simulink model "FH_SS"  (R2018b)
settings: Solver=ode5  StartTime=0.0  StopTime=N*Tb  FixedStep=Tsampling  RelTol=1e-3
values from neighbouring files (symbols this model uses):
  Eb = 2    [FH_Script.m]
  Tb = 1/100    (= 0.01)    [FH_Script.m]
  Tc = Tb/(MultPer*Nchips)    (= 0.000285714285714)    [FH_Script.m]
libraries: dsparch4 x5, commsynccomp2 x4, commrandsrc3 x1, simulink x1
settings Model: Creator=lukit  LastModifiedBy=lukit

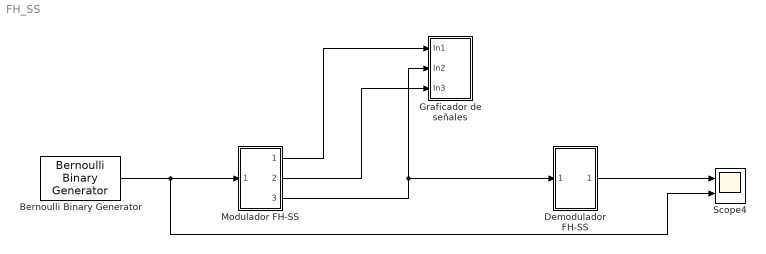
== system FH_SS ==
  Bernoulli Binary Generator : commrandsrc3/Bernoulli Binary Generator  ProbabilityOfZero=0.5  SeedSource=Auto  Seed=0  SampleTime=Tb  SamplesPerFrame=1  OutputDataType=double  SimulateUsing=Interpreted execution
  Demodulador FH-SS : Subsystem
  Graficador de señales : Subsystem
  Modulador FH-SS : Subsystem
  Scope4 : Scope  NumInputPorts=2
  wires:
  Modulador FH-SS/3(Out3) -> Demodulador FH-SS/1(In1), Graficador de señales/2(In2)
  Bernoulli Binary Generator/1 -> Scope4/2, Modulador FH-SS/1(In1)
  Modulador FH-SS/1(Out1) -> Graficador de señales/1(In1)
  Modulador FH-SS/2(Out2) -> Graficador de señales/3(In3)
  Demodulador FH-SS/1(Out1) -> Scope4/1

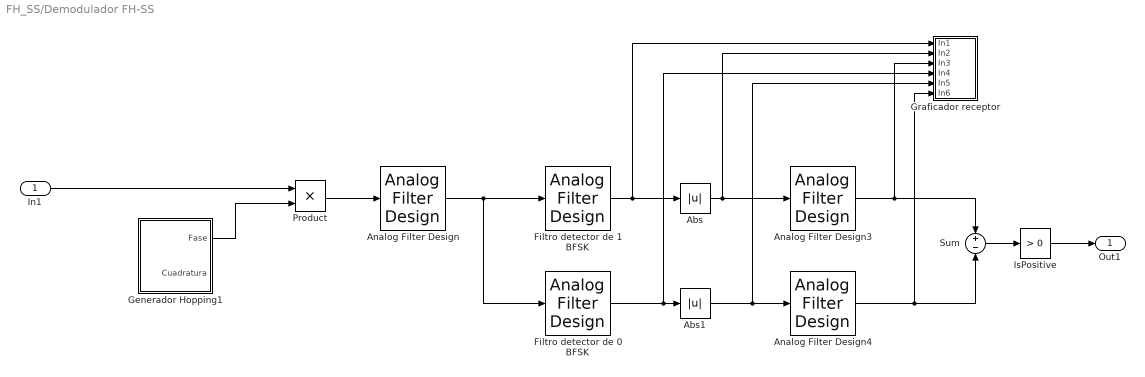
== system FH_SS/Demodulador FH-SS ==
  In1 : Inport
  Abs : Abs
  Abs1 : Abs
  Analog Filter Design : dsparch4/Analog Filter Design  method=Butterworth  filttype=Bandpass  N=8  Wlo=2*pi*(2*(1/Tc) - (1/Tc))  Whi=2*pi*(4*(1/Tc) +(1/Tc))  Rp=2  Rs=40
  Analog Filter Design3 : dsparch4/Analog Filter Design  method=Butterworth  filttype=Lowpass  N=8  Wlo=2*pi*((1/Tc))  Whi=2*pi*((2*(1/Tc)) +(1/Tc))  Rp=2  Rs=40
  Analog Filter Design4 : dsparch4/Analog Filter Design  method=Butterworth  filttype=Lowpass  N=8  Wlo=2*pi*((1/Tc))  Whi=2*pi*((2*(1/Tc)) +(1/Tc))  Rp=2  Rs=40
  Filtro detector de 0 BFSK : dsparch4/Analog Filter Design  method=Butterworth  filttype=Bandpass  N=8  Wlo=2*pi*((4*(1/Tc)) - (1/Tc))  Whi=2*pi*((4*(1/Tc)) +(1/Tc))  Rp=2  Rs=40
  Filtro detector de 1 BFSK : dsparch4/Analog Filter Design  method=Butterworth  filttype=Bandpass  N=8  Wlo=2*pi*((2*(1/Tc)) - (1/Tc))  Whi=2*pi*((2*(1/Tc)) +(1/Tc))  Rp=2  Rs=40
  Generador Hopping1 : Subsystem
  Graficador receptor : Subsystem
  IsPositive : simulink/Logic and Bit Operations/Compare To Zero  relop=>  OutDataTypeStr=boolean
  Product : Product
  Sum : Sum  Inputs=+-
  Out1 : Outport
  wires:
  Product/1 -> Analog Filter Design/1
  Analog Filter Design3/1 -> Sum/1, Graficador receptor/3(In3)
  Abs/1 -> Analog Filter Design3/1, Graficador receptor/2(In2)
  Filtro detector de 1 BFSK/1 -> Abs/1, Graficador receptor/1(In1)
  Generador Hopping1/1(Fase) -> Product/2
  Analog Filter Design/1 -> Filtro detector de 0 BFSK/1, Filtro detector de 1 BFSK/1
  Analog Filter Design4/1 -> Sum/2, Graficador receptor/6(In6)
  Filtro detector de 0 BFSK/1 -> Graficador receptor/4(In4), Abs1/1
  Abs1/1 -> Graficador receptor/5(In5), Analog Filter Design4/1
  In1/1 -> Product/1
  Sum/1 -> IsPositive/1
  IsPositive/1 -> Out1/1

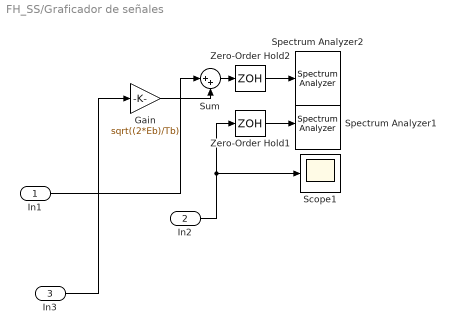
== system FH_SS/Graficador de señales ==
  In1 : Inport
  In2 : Inport  Port=2
  In3 : Inport  Port=3
  Gain : Gain  Gain=sqrt((2*Eb)/Tb)
  Scope1 : Scope
  Spectrum Analyzer1 : SpectrumAnalyzer
  Spectrum Analyzer2 : SpectrumAnalyzer
  Sum : Sum  Inputs=|++
  Zero-Order Hold1 : ZeroOrderHold  SampleTime=-1
  Zero-Order Hold2 : ZeroOrderHold  SampleTime=-1
  wires:
  In1/1 -> Sum/1
  Zero-Order Hold1/1 -> Spectrum Analyzer1/1
  Zero-Order Hold2/1 -> Spectrum Analyzer2/1
  In2/1 -> Scope1/1, Zero-Order Hold1/1
  Sum/1 -> Zero-Order Hold2/1
  In3/1 -> Gain/1
  Gain/1 -> Sum/2

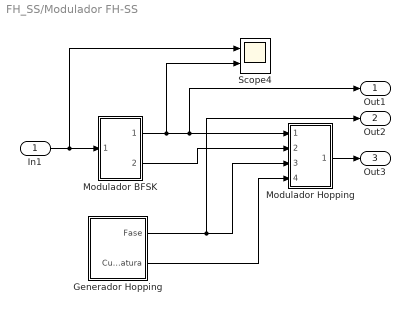
== system FH_SS/Modulador FH-SS ==
  In1 : Inport
  Generador Hopping : Subsystem
  Modulador BFSK : Subsystem
  Modulador Hopping : Subsystem
  Scope4 : Scope  NumInputPorts=2
  Out1 : Outport
  Out2 : Outport  Port=2
  Out3 : Outport  Port=3
  wires:
  Modulador BFSK/2(Out2) -> Modulador Hopping/2(In2)
  Modulador BFSK/1(Out1) -> Scope4/2, Out1/1, Modulador Hopping/1(In1)
  Generador Hopping/1(Fase) -> Out2/1, Modulador Hopping/3(In3)
  In1/1 -> Scope4/1, Modulador BFSK/1(In1)
  Modulador Hopping/1(Out1) -> Out3/1
  Generador Hopping/2(Cuadratura) -> Modulador Hopping/4(In4)

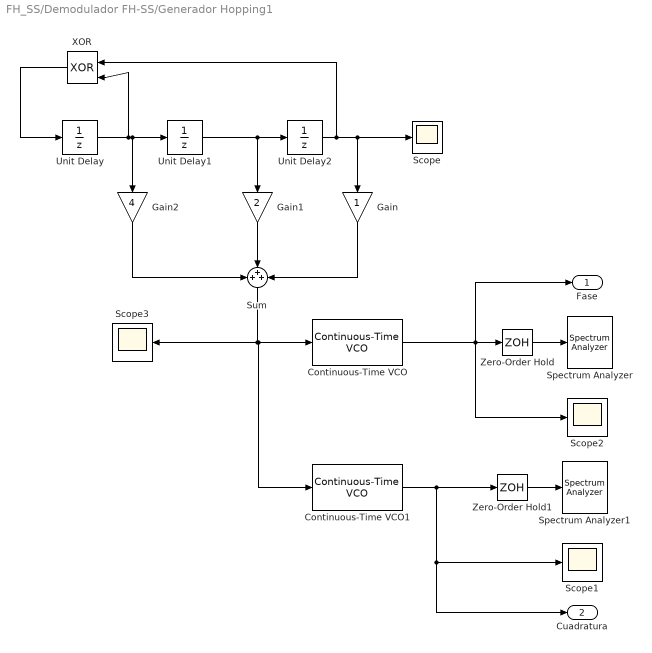
== system FH_SS/Demodulador FH-SS/Generador Hopping1 ==
  Continuous-Time VCO : commsynccomp2/Continuous-Time VCO  Ac=1  Fc=1/Tc  Kc=FrecSignal  Ph=0
      settings: SourceProductName=Communications System Toolbox  SourceProductBaseCode=CM
  Continuous-Time VCO1 : commsynccomp2/Continuous-Time VCO  Ac=1  Fc=1/Tc  Kc=FrecSignal  Ph=pi/2
      settings: SourceProductName=Communications System Toolbox  SourceProductBaseCode=CM
  Gain : Gain
  Gain1 : Gain  Gain=2
  Gain2 : Gain  Gain=4
  Scope{,1..3} (4 alike) : Scope
  Spectrum Analyzer : SpectrumAnalyzer
  Spectrum Analyzer1 : SpectrumAnalyzer
  Sum : Sum  Inputs=+++  OutDataTypeStr=double
  Unit Delay : UnitDelay  SampleTime=Tc
  Unit Delay1 : UnitDelay  SampleTime=Tc
  Unit Delay2 : UnitDelay  InitialCondition=1  SampleTime=Tc
  XOR : Logic  Operator=XOR  IconShape=distinctive  AllPortsSameDT=off  OutDataTypeStr=boolean
  Zero-Order Hold : ZeroOrderHold  SampleTime=-1
  Zero-Order Hold1 : ZeroOrderHold  SampleTime=-1
  Fase : Outport
  Cuadratura : Outport  Port=2
  wires:
  Gain2/1 -> Sum/1
  Unit Delay/1 -> XOR/2, Gain2/1, Unit Delay1/1
  Sum/1 -> Continuous-Time VCO1/1, Continuous-Time VCO/1, Scope3/1
  XOR/1 -> Unit Delay/1
  Unit Delay1/1 -> Gain1/1, Unit Delay2/1
  Unit Delay2/1 -> Gain/1, Scope/1, XOR/1
  Zero-Order Hold/1 -> Spectrum Analyzer/1
  Gain1/1 -> Sum/2
  Gain/1 -> Sum/3
  Continuous-Time VCO/1 -> Scope2/1, Zero-Order Hold/1, Fase/1
  Continuous-Time VCO1/1 -> Zero-Order Hold1/1, Cuadratura/1, Scope1/1
  Zero-Order Hold1/1 -> Spectrum Analyzer1/1

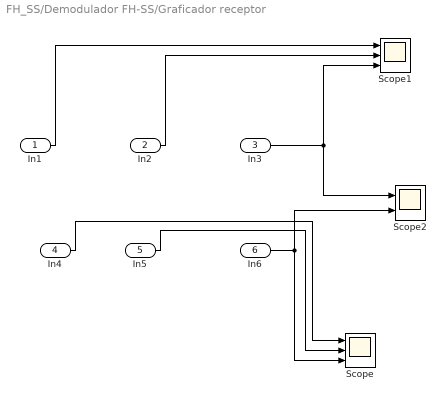
== system FH_SS/Demodulador FH-SS/Graficador receptor ==
  In1 : Inport
  In2 : Inport  Port=2
  In3 : Inport  Port=3
  In4 : Inport  Port=4
  In5 : Inport  Port=5
  In6 : Inport  Port=6
  Scope : Scope  NumInputPorts=3
  Scope1 : Scope  NumInputPorts=3
  Scope2 : Scope  NumInputPorts=2
  wires:
  In6/1 -> Scope2/2, Scope/3
  In3/1 -> Scope1/3, Scope2/1
  In2/1 -> Scope1/2
  In4/1 -> Scope/1
  In1/1 -> Scope1/1
  In5/1 -> Scope/2

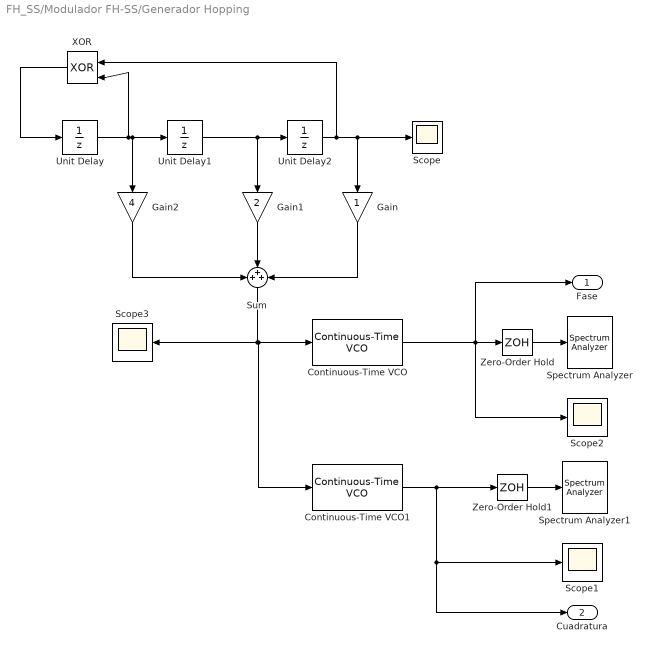
== system FH_SS/Modulador FH-SS/Generador Hopping ==
  Continuous-Time VCO : commsynccomp2/Continuous-Time VCO  Ac=1  Fc=1/Tc  Kc=FrecSignal  Ph=0
      settings: SourceProductName=Communications System Toolbox  SourceProductBaseCode=CM
  Continuous-Time VCO1 : commsynccomp2/Continuous-Time VCO  Ac=1  Fc=1/Tc  Kc=FrecSignal  Ph=pi/2
      settings: SourceProductName=Communications System Toolbox  SourceProductBaseCode=CM
  Gain : Gain
  Gain1 : Gain  Gain=2
  Gain2 : Gain  Gain=4
  Scope{,1..3} (4 alike) : Scope
  Spectrum Analyzer : SpectrumAnalyzer
  Spectrum Analyzer1 : SpectrumAnalyzer
  Sum : Sum  Inputs=+++  OutDataTypeStr=double
  Unit Delay : UnitDelay  SampleTime=Tc
  Unit Delay1 : UnitDelay  SampleTime=Tc
  Unit Delay2 : UnitDelay  InitialCondition=1  SampleTime=Tc
  XOR : Logic  Operator=XOR  IconShape=distinctive  AllPortsSameDT=off  OutDataTypeStr=boolean
  Zero-Order Hold : ZeroOrderHold  SampleTime=-1
  Zero-Order Hold1 : ZeroOrderHold  SampleTime=-1
  Fase : Outport
  Cuadratura : Outport  Port=2
  wires:
  Gain2/1 -> Sum/1
  Unit Delay/1 -> XOR/2, Gain2/1, Unit Delay1/1
  Sum/1 -> Continuous-Time VCO1/1, Continuous-Time VCO/1, Scope3/1
  XOR/1 -> Unit Delay/1
  Unit Delay1/1 -> Gain1/1, Unit Delay2/1
  Unit Delay2/1 -> Gain/1, Scope/1, XOR/1
  Zero-Order Hold/1 -> Spectrum Analyzer/1
  Gain1/1 -> Sum/2
  Gain/1 -> Sum/3
  Continuous-Time VCO/1 -> Scope2/1, Zero-Order Hold/1, Fase/1
  Continuous-Time VCO1/1 -> Zero-Order Hold1/1, Cuadratura/1, Scope1/1
  Zero-Order Hold1/1 -> Spectrum Analyzer1/1

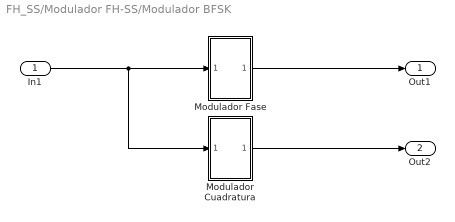
== system FH_SS/Modulador FH-SS/Modulador BFSK ==
  In1 : Inport
  Modulador Cuadratura : Subsystem
  Modulador Fase : Subsystem
  Out1 : Outport
  Out2 : Outport  Port=2
  wires:
  In1/1 -> Modulador Cuadratura/1(In1), Modulador Fase/1(In1)
  Modulador Cuadratura/1(Out1) -> Out2/1
  Modulador Fase/1(Out1) -> Out1/1

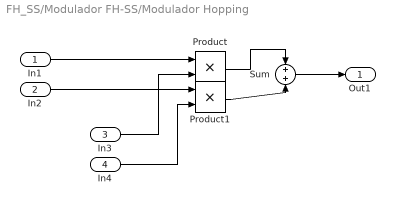
== system FH_SS/Modulador FH-SS/Modulador Hopping ==
  In1 : Inport
  In2 : Inport  Port=2
  In3 : Inport  Port=3
  In4 : Inport  Port=4
  Product : Product
  Product1 : Product
  Sum : Sum
  Out1 : Outport
  wires:
  Product1/1 -> Sum/2
  Sum/1 -> Out1/1
  Product/1 -> Sum/1
  In2/1 -> Product1/1
  In1/1 -> Product/1
  In3/1 -> Product/2
  In4/1 -> Product1/2

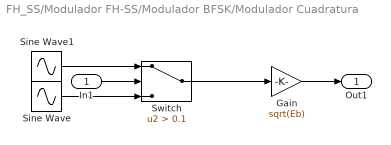
== system FH_SS/Modulador FH-SS/Modulador BFSK/Modulador Cuadratura ==
  In1 : Inport
  Gain : Gain  Gain=sqrt(Eb)
  Sine Wave : Sin  Amplitude=sqrt(2/Tb)  Frequency=2*pi*(4*(1/Tc))  SampleTime=0
  Sine Wave1 : Sin  Amplitude=sqrt(2/Tb)  Frequency=2*pi*(2*(1/Tc))  SampleTime=0
  Switch : Switch  Criteria=u2 > Threshold  Threshold=0.1
  Out1 : Outport
  wires:
  Sine Wave1/1 -> Switch/1
  Sine Wave/1 -> Switch/3
  Switch/1 -> Gain/1
  In1/1 -> Switch/2
  Gain/1 -> Out1/1

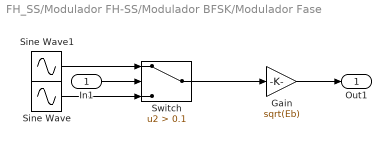
== system FH_SS/Modulador FH-SS/Modulador BFSK/Modulador Fase ==
  In1 : Inport
  Gain : Gain  Gain=sqrt(Eb)
  Sine Wave : Sin  Amplitude=sqrt(2/Tb)  Frequency=2*pi*(4*(1/Tc))  Phase=pi/2  SampleTime=0
  Sine Wave1 : Sin  Amplitude=sqrt(2/Tb)  Frequency=2*pi*(2*(1/Tc))  Phase=pi/2  SampleTime=0
  Switch : Switch  Criteria=u2 > Threshold  Threshold=0.1
  Out1 : Outport
  wires:
  Sine Wave1/1 -> Switch/1
  Sine Wave/1 -> Switch/3
  Switch/1 -> Gain/1
  In1/1 -> Switch/2
  Gain/1 -> Out1/1
